simulink model "updated"  (R2024b)
settings: Solver=ode23tb  StartTime=0.0  StopTime=150  RelTol=1e-3
libraries: slpidlib x1
settings Model: Creator=ITER  LastModifiedBy=naina
settings RTWCC: GPUComputeCapability=3.5

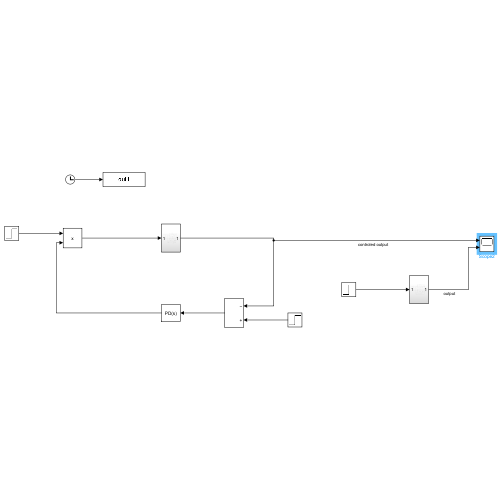
[thumbnail: Simulink's stored preview of the top-level diagram]
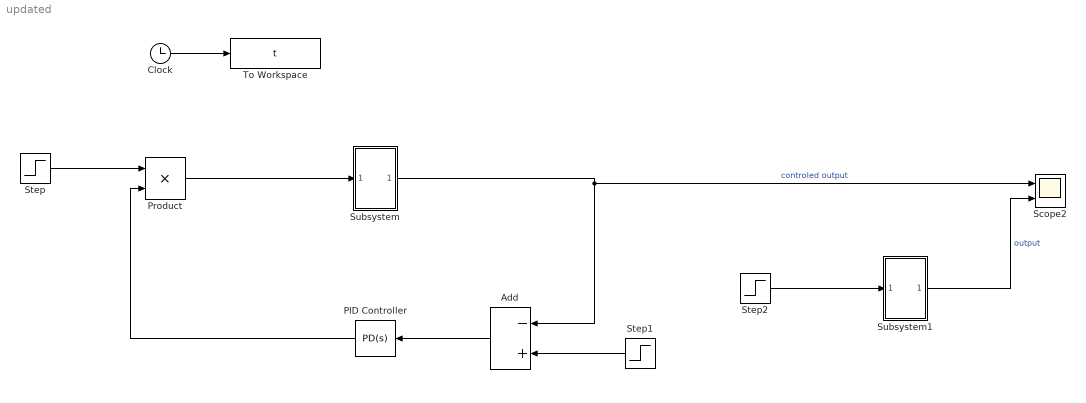
== system updated ==
  Add : Sum  Inputs=-+
  Clock : Clock
  PID Controller : slpidlib/PID Controller  Controller=PD  Form=Parallel  TimeDomain=Continuous-time  UseExternalTs=off  SampleTime=-1  IntegratorMethod=Forward Euler  FilterMethod=Forward Euler  ControllerParametersSource=internal  P=0.0011  I=1  UseKiTs=off  D=0.001  UseExternalDerivativeSource=off  N=100  UseFilter=on  TunerSelectOption=Transfer Function Based (PID Tuner App)  InitialConditionSource=internal  InitialConditionForIntegrator=0  InitialConditionForFilter=0  DifferentiatorICPrevScaledInput=0  ExternalReset=none  TrackingMode=off  Kt=1  LimitOutput=off  SatLimitsSource=internal  UpperSaturationLimit=inf  LowerSaturationLimit=-inf  LinearizeAsGain=on  AntiWindupMode=none  Kb=1  LimitIntegrator=off  UpperIntegratorSaturationLimit=inf  LowerIntegratorSaturationLimit=-inf  POutMin=[]  POutMax=[]  IOutMin=[]  IOutMax=[]  DOutMin=[]  DOutMax=[]  NOutMin=[]  NOutMax=[]  SumOutMin=[]  SumOutMax=[]  SaturationOutMin=[]  SaturationOutMax=[]  PParamMin=[]  PParamMax=[]  IParamMin=[]  IParamMax=[]  DParamMin=[]  DParamMax=[]  NParamMin=[]  NParamMax=[]  KbParamMin=[]  KbParamMax=[]  KtParamMin=[]  KtParamMax=[]  KbOutMin=[]  KbOutMax=[]  KtOutMin=[]  KtOutMax=[]  IntegratorOutMin=[]  IntegratorOutMax=[]  FilterOutMin=[]  FilterOutMax=[]  SumI1OutMin=[]  SumI1OutMax=[]  SumI2OutMin=[]  SumI2OutMax=[]  SumI3OutMin=[]  SumI3OutMax=[]  SumI4OutMin=[]  SumI4OutMax=[]  SumDOutMin=[]  SumDOutMax=[]  DifferentiatorOutMin=[]  DifferentiatorOutMax=[]  FilterDiffOutCoefMin=[]  FilterDiffOutCoefMax=[]  ReciprocalOutMin=[]  ReciprocalOutMax=[]  SumDenOutMin=[]  SumDenOutMax=[]  SumNumOutMin=[]  SumNumOutMax=[]  DivideOutMin=[]  DivideOutMax=[]  UdiffTsProdOutMin=[]  UdiffTsProdOutMax=[]  NTsProdOutMin=[]  NTsProdOutMax=[]  UintegralTsProdOutMin=[]  UintegralTsProdOutMax=[]  UngainTsProdOutMin=[]  UngainTsProdOutMax=[]  ClampingZeroOutDataTypeStr=Inherit: Inherit via back propagation  ClampingZeroOutMin=[]  ClampingZeroOutMax=[]  FilterDenConstantOutDataTypeStr=Inherit: Inherit via back propagation  FilterDenConstantOutMin=[]  FilterDenConstantOutMax=[]  PCopyOutDataTypeStr=Inherit: Inherit via back propagation  PCopyOutMin=[]  PCopyOutMax=[]  NCopyOutDataTypeStr=Inherit: Inherit via back propagation  NCopyOutMin=[]  NCopyOutMax=[]  IntegratorContinuousStateAttributes=''  IntegratorStateMustResolveToSignalObject=off  IntegratorRTWStateStorageClass=Auto  FilterContinuousStateAttributes=''  FilterStateMustResolveToSignalObject=off  FilterRTWStateStorageClass=Auto  ParallelPVariant=InternalParameters  IdealPVariant=Disabled  IVariant=Disabled  DVariant=InternalParameters  IntegratorVariant=Disabled  SatVariant=Disabled  AWVariant=Disabled  PCopyVariant=Disabled  TRVariant=Disabled  FdbkBlocksVariant=Forward  IdealPFdbkVariant=Disabled  SatFdbkVariant=Disabled  DerivativeFilterVariant=ContFilter  NVariant=InternalParameters  NCopyVariant=Disabled  FilterICVariant=InternalICsFilter  IntegratorICVariant=Disabled  ExternalResetVariant=Disabled  TRSumVariant=Passthrough  SumFdbkVariant=Disabled  SumVariant=Sum_PD  TsampFilterVariant=InternalTs  TsampNgainVariant=Passthrough  TsampIntegralVariant=Disabled_SignalSpec  ExternalSaturationOutDataTypeStr=Inherit: Same as second input  DerivativeSourceVariant=ErrorSignal  PreIntVariant=InternalPreInt
  Product : Product
  Scope2 : Scope  NumInputPorts=2
  Step : Step  Time=0  SampleTime=0
  Step1 : Step  Time=0  SampleTime=0
  Step2 : Step  SampleTime=0
  Subsystem : Subsystem
  Subsystem1 : Subsystem
  To Workspace : ToWorkspace  VariableName=t  SaveFormat=Timeseries  SampleTime=-1
  wires:
  Subsystem/1(Out1) -> Scope2/1, Add/1  "controled output"
  Step/1 -> Product/1
  PID Controller/1 -> Product/2
  Add/1 -> PID Controller/1
  Step1/1 -> Add/2
  Product/1 -> Subsystem/1(In1)
  Clock/1 -> To Workspace/1
  Step2/1 -> Subsystem1/1(In1)
  Subsystem1/1(Out1) -> Scope2/2  "output"

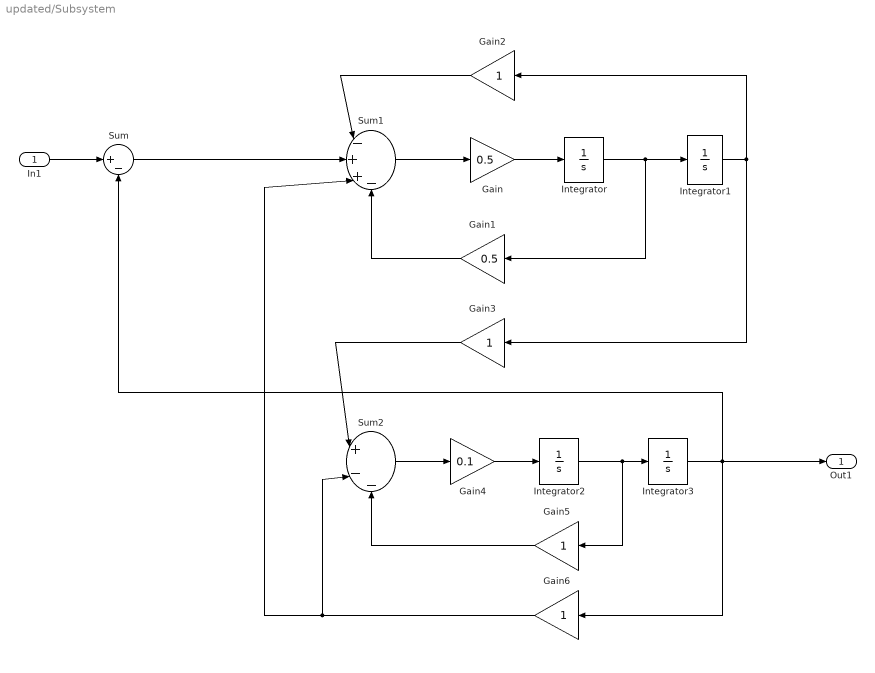
== system updated/Subsystem ==
  In1 : Inport
  Gain : Gain  Gain=0.5
  Gain1 : Gain  Gain=0.5
  Gain{2..3,5..6} (4 alike) : Gain
  Gain4 : Gain  Gain=0.1
  Integrator{,1..3} (4 alike) : Integrator
  Sum : Sum  Inputs=|+-
  Sum1 : Sum  Inputs=|-++-
  Sum2 : Sum  Inputs=|+--
  Out1 : Outport
  wires:
  Gain6/1 -> Sum2/2, Sum1/3
  Sum/1 -> Sum1/2
  Integrator2/1 -> Gain5/1, Integrator3/1
  Gain4/1 -> Integrator2/1
  Integrator/1 -> Gain1/1, Integrator1/1
  Gain5/1 -> Sum2/3
  Integrator3/1 -> Out1/1, Sum/2, Gain6/1
  Integrator1/1 -> Gain2/1, Gain3/1
  Gain1/1 -> Sum1/4
  Sum2/1 -> Gain4/1
  Gain2/1 -> Sum1/1
  Gain/1 -> Integrator/1
  Sum1/1 -> Gain/1
  Gain3/1 -> Sum2/1
  In1/1 -> Sum/1

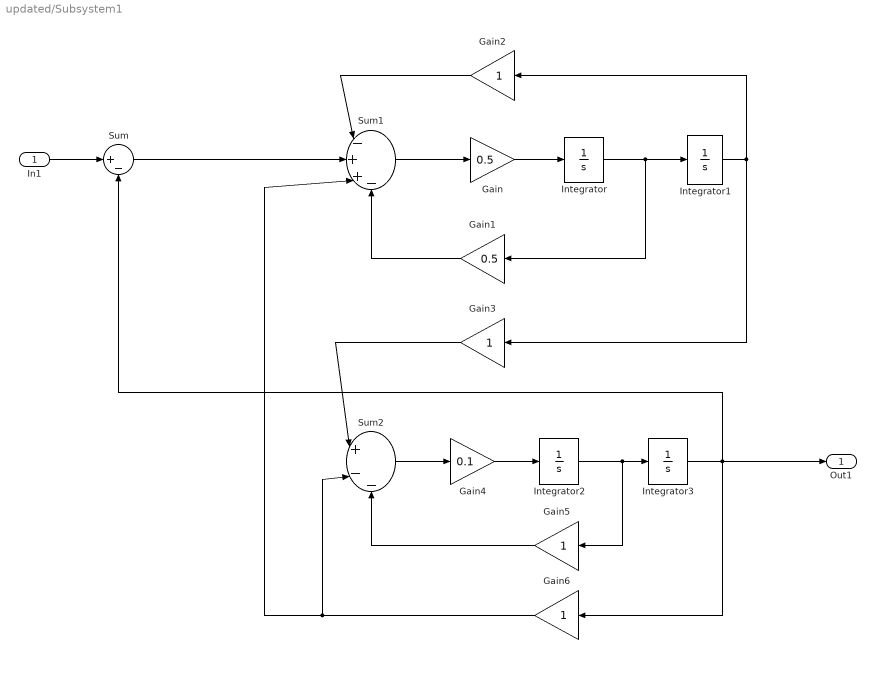
== system updated/Subsystem1 ==
  In1 : Inport
  Gain : Gain  Gain=0.5
  Gain1 : Gain  Gain=0.5
  Gain{2..3,5..6} (4 alike) : Gain
  Gain4 : Gain  Gain=0.1
  Integrator{,1..3} (4 alike) : Integrator
  Sum : Sum  Inputs=|+-
  Sum1 : Sum  Inputs=|-++-
  Sum2 : Sum  Inputs=|+--
  Out1 : Outport
  wires:
  Gain6/1 -> Sum2/2, Sum1/3
  Sum/1 -> Sum1/2
  Integrator2/1 -> Gain5/1, Integrator3/1
  Gain4/1 -> Integrator2/1
  Integrator/1 -> Gain1/1, Integrator1/1
  Gain5/1 -> Sum2/3
  Integrator3/1 -> Out1/1, Sum/2, Gain6/1
  Integrator1/1 -> Gain2/1, Gain3/1
  Gain1/1 -> Sum1/4
  Sum2/1 -> Gain4/1
  Gain2/1 -> Sum1/1
  Gain/1 -> Integrator/1
  Sum1/1 -> Gain/1
  Gain3/1 -> Sum2/1
  In1/1 -> Sum/1
